simulink library "simple_moving_average_filter"  (R2025b)
settings: Solver=VariableStepAuto  StartTime=0.0  StopTime=10.0  RelTol=1e-3
undefined symbols (not defined in the file): ts_afe
libraries: simulink x1
settings Model: Creator=dbagn  LastModifiedBy=dbagn

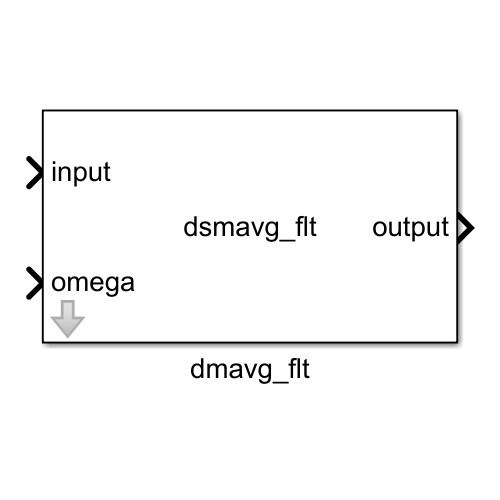
[thumbnail: Simulink's stored preview of the top-level diagram]
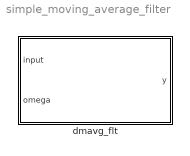
== system simple_moving_average_filter ==
  dmavg_flt : Subsystem  mask{ts=ts_afe}
      mask prompts: ts "sampling time (s)"
      mask Display:
      | disp('dsmavg_flt');
      | port_label('input', 1, 'input');
      | port_label('input', 2, 'omega');
      | port_label('output', 1, 'output');

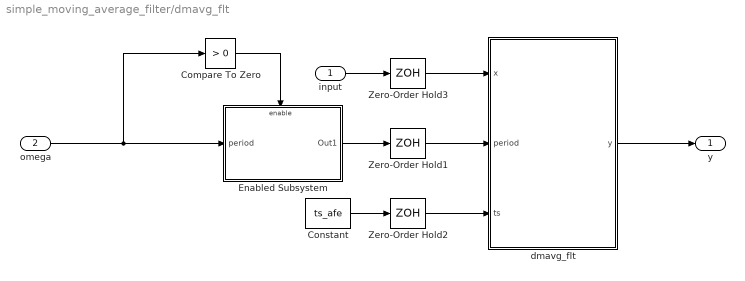
== system simple_moving_average_filter/dmavg_flt ==
  input : Inport
  omega : Inport  Port=2
  Compare To Zero : simulink/Logic and Bit Operations/Compare To Zero  relop=>  OutDataTypeStr=boolean
  Constant : Constant  Value=ts_afe
  Enabled Subsystem : Subsystem  TreatAsAtomicUnit=on
  Zero-Order Hold1 : ZeroOrderHold  SampleTime=-1
  Zero-Order Hold2 : ZeroOrderHold  SampleTime=-1
  Zero-Order Hold3 : ZeroOrderHold  SampleTime=-1
  dmavg_flt : MATLAB Function  TreatAsAtomicUnit=on
  y : Outport
  wires:
  dmavg_flt/1(y) -> y/1
  Constant/1 -> Zero-Order Hold2/1
  input/1 -> Zero-Order Hold3/1
  Compare To Zero/1 -> Enabled Subsystem/Enable
  Enabled Subsystem/1(Out1) -> Zero-Order Hold1/1
  omega/1 -> Compare To Zero/1, Enabled Subsystem/1(period)
  Zero-Order Hold3/1 -> dmavg_flt/1(x)
  Zero-Order Hold1/1 -> dmavg_flt/2(period)
  Zero-Order Hold2/1 -> dmavg_flt/3(ts)

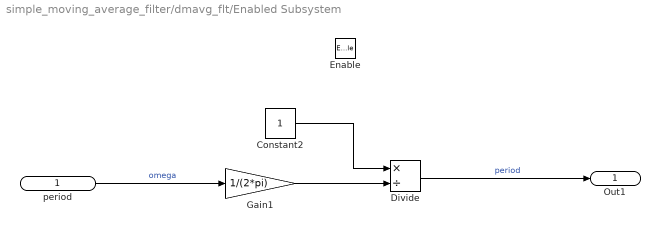
== system simple_moving_average_filter/dmavg_flt/Enabled Subsystem ==
  period : Inport
  Enable : EnablePort
  Constant2 : Constant
  Divide : Product  Inputs=*/
  Gain1 : Gain  Gain=1/(2*pi)
  Out1 : Outport
  wires:
  Constant2/1 -> Divide/1
  period/1 -> Gain1/1  "omega"
  Gain1/1 -> Divide/2
  Divide/1 -> Out1/1  "period"

== matlab function simple_moving_average_filter/dmavg_flt/dmavg_flt ==
  data: x input; y output; period input; ts input
function y = dmavg_flt(x, period, ts)
    persistent buffer idx length_period sum_buffer Nmax

    Nmax = 1600;

    if isempty(buffer)
        buffer = zeros(1, Nmax);
        idx = 1;
        sum_buffer = 0;
    end

    length_period = floor(period / ts) + 1;

    % Compute index of oldest sample (circular buffer)
    old_idx = mod(idx - length_period - 1, Nmax) + 1;
    xn = buffer(old_idx);

    % Update sum and buffer
    sum_buffer = sum_buffer - xn + x;
    buffer(idx) = x;

    % Compute average
    y = sum_buffer / length_period;

    % Advance circular index
    idx = mod(idx, Nmax) + 1;
end
